simulink model "rele_b1"  (R2017a)
settings: Solver=FixedStepAuto  StartTime=0.0  StopTime=100  FixedStep=0.03  RelTol=1e-3
settings Model: Creator=bruno  LastModifiedBy=LuísFelipeVieiraSilv
settings DataIOCC: LimitDataPoints=on  SaveFormat=Array
settings OptimizationCC: BlockReduction=off  BooleanDataType=off  LifeSpan=inf
settings DebuggingCC: SaveWithParameterizedLinksMsg=none  UnderspecifiedInitializationDetection=Classic  MergeDetectMultiDrivingBlocksExec=none  SignalResolutionControl=TryResolveAllWithWarning  SFUnexpectedBacktrackingDiag=warning  SFNoUnconditionalDefaultTransitionDiag=warning  SFExecutionAtInitializationDiag=none
settings HardwareCC: ProdBitPerPointer=32  ProdBitPerSizeT=32  ProdBitPerPtrDiffT=32  ProdLargestAtomicFloat=None  ProdIntDivRoundTo=Undefined  ProdEndianess=Unspecified  ProdWordSize=32  ProdHWDeviceType=32-bit Generic  TargetUnknown=on
settings ModelReferenceCC: PropagateSignalLabelsOutOfModel=off
settings GRTTargetCC: TargetLangStandard=C89/C90 (ANSI)  GeneratePreprocessorConditionals=Disable all
settings ConfigComp: CovMetricSettings=dw  CovHtmlReporting=on  CovSaveCumulativeToWorkspaceVar=on  CovSaveSingleToWorkspaceVar=on  CovExternalEMLEnable=off  CovSFcnEnable=off

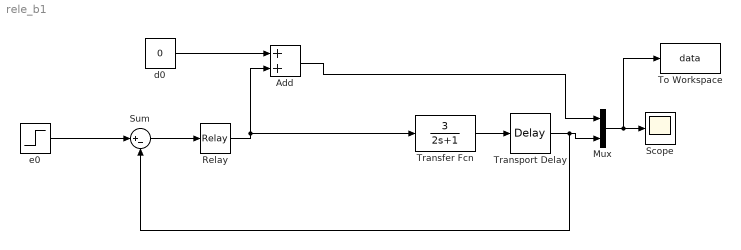
== system rele_b1 ==
  Add : Sum
  Mux : Mux  Inputs=2
  Relay : Relay  OnSwitchValue=0.9  OffSwitchValue=-0.9  OnOutputValue=2.5  OffOutputValue=-0.5
  Scope : Scope
  Sum : Sum  Inputs=|+-
  To Workspace : ToWorkspace  VariableName=data  SampleTime=-1
  Transfer Fcn : TransferFcn  Numerator=[3]  Denominator=[2 1]
  Transport Delay : TransportDelay  DelayTime=0.1
  d0 : Constant  Value=0
  "e0 " : Step  Time=0  SampleTime=0
  wires:
  Mux/1 -> To Workspace/1, Scope/1
  Sum/1 -> Relay/1
  d0/1 -> Add/1
  Relay/1 -> Transfer Fcn/1, Add/2
  Add/1 -> Mux/1
  "e0 "/1 -> Sum/1
  Transfer Fcn/1 -> Transport Delay/1
  Transport Delay/1 -> Sum/2, Mux/2
